simulink model "sensor_model"  (R2018a)
settings: Solver=ode15s  StartTime=0.0  StopTime=200  RelTol=1e-3
libraries: simulink x3
settings Model: Creator=cory0  LastModifiedBy=sanjana

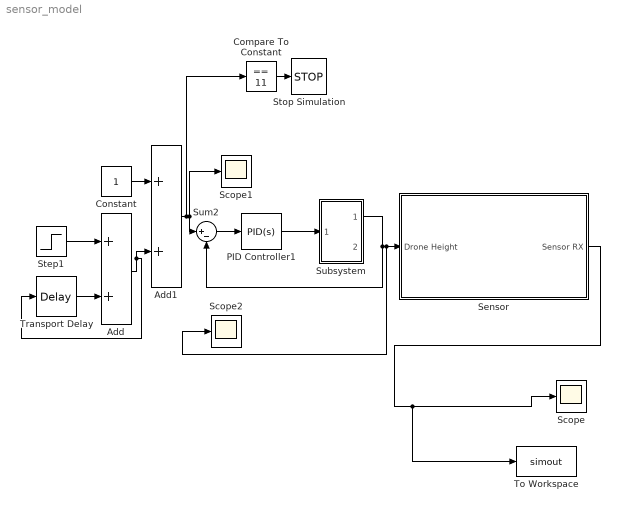
== system sensor_model ==
  Add : Sum
  Add1 : Sum
  Compare To Constant : simulink/Logic and Bit Operations/Compare To Constant  relop===  const=11  OutDataTypeStr=boolean
  Constant : Constant
  PID Controller1 : simulink/Continuous/PID Controller  Controller=PID  TimeDomain=Continuous-time  SampleTime=-1  IntegratorMethod=Forward Euler  FilterMethod=Forward Euler  Form=Parallel  UseFilter=on  ControllerParametersSource=internal  P=85  I=0  D=85  N=10  InitialConditionSource=internal  InitialConditionForIntegrator=0  InitialConditionForFilter=0  ExternalReset=none  LimitOutput=off  UpperSaturationLimit=inf  LowerSaturationLimit=-inf  LinearizeAsGain=on  AntiWindupMode=none  Kb=1  TrackingMode=off  Kt=1  PParamMin=[]  PParamMax=[]  IParamMin=[]  IParamMax=[]  DParamMin=[]  DParamMax=[]  NParamMin=[]  NParamMax=[]  KbParamMin=[]  KbParamMax=[]  KtParamMin=[]  KtParamMax=[]  POutMin=[]  POutMax=[]  IOutMin=[]  IOutMax=[]  DOutMin=[]  DOutMax=[]  NOutMin=[]  NOutMax=[]  KbOutMin=[]  KbOutMax=[]  KtOutMin=[]  KtOutMax=[]  IntegratorOutMin=[]  IntegratorOutMax=[]  FilterOutMin=[]  FilterOutMax=[]  SumOutMin=[]  SumOutMax=[]  SumI1OutMin=[]  SumI1OutMax=[]  SumI2OutMin=[]  SumI2OutMax=[]  SumI3OutMin=[]  SumI3OutMax=[]  SumDOutMin=[]  SumDOutMax=[]  SaturationOutMin=[]  SaturationOutMax=[]  IntegratorContinuousStateAttributes=''  IntegratorStateMustResolveToSignalObject=off  IntegratorRTWStateStorageClass=Auto  FilterContinuousStateAttributes=''  FilterStateMustResolveToSignalObject=off  FilterRTWStateStorageClass=Auto  DifferentiatorICPrevScaledInput=0  DifferentiatorOutMin=[]  DifferentiatorOutMax=[]  FilterDiffOutCoefMin=[]  FilterDiffOutCoefMax=[]  SumDenOutMin=[]  SumDenOutMax=[]  SumNumOutMin=[]  SumNumOutMax=[]  ReciprocalOutMin=[]  ReciprocalOutMax=[]  DivideOutMin=[]  DivideOutMax=[]  TunerSelectOption=Transfer Function Based (PID Tuner App)
  Scope : Scope
  Scope1 : Scope
  Scope2 : Scope
  Sensor : Subsystem
  Step1 : Step  Time=15  SampleTime=0
  Stop Simulation : Stop
  Subsystem : Subsystem
  Sum2 : Sum  Inputs=|+-
  To Workspace : ToWorkspace  VariableName=simout  SampleTime=0.005
  Transport Delay : TransportDelay  DelayTime=20
  wires:
  Constant/1 -> Add1/1
  Subsystem/1(Out1) -> Scope2/1, Sensor/1(Drone Height), Sum2/2
  PID Controller1/1 -> Subsystem/1(In1)
  Sum2/1 -> PID Controller1/1
  Transport Delay/1 -> Add/2
  Step1/1 -> Add/1
  Add1/1 -> Compare To Constant/1, Scope1/1, Sum2/1
  Add/1 -> Transport Delay/1, Add1/2
  Compare To Constant/1 -> Stop Simulation/1
  Sensor/1(Sensor RX) -> To Workspace/1, Scope/1

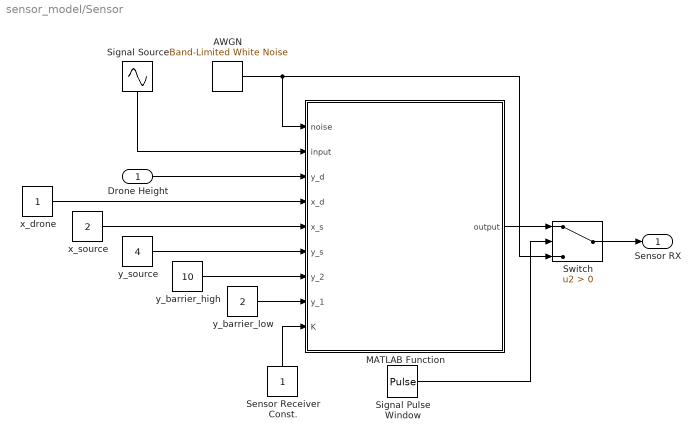
== system sensor_model/Sensor ==
  Drone Height : Inport
  AWGN : simulink/Sources/Band-Limited White Noise  Cov=[0.00001]  Ts=0.0005  seed=[23340]
  MATLAB Function : MATLAB Function  TreatAsAtomicUnit=on
  Sensor Receiver Const. : Constant
  Signal Source : Sin  Amplitude=10  Frequency=6.2831853  SampleTime=0
  Signal Pulse Window : DiscretePulseGenerator  PulseType=Time based  Period=20  PulseWidth=75
  Switch : Switch  Criteria=u2 > Threshold
  x_drone : Constant
  x_source : Constant  Value=2
  y_barrier_high : Constant  Value=10
  y_barrier_low : Constant  Value=2
  y_source : Constant  Value=4
  Sensor RX : Outport
  wires:
  Sensor Receiver Const./1 -> MATLAB Function/9(K)
  Signal Source/1 -> MATLAB Function/2(input)
  Signal Pulse Window/1 -> Switch/2
  y_source/1 -> MATLAB Function/6(y_s)
  y_barrier_low/1 -> MATLAB Function/8(y_1)
  x_drone/1 -> MATLAB Function/4(x_d)
  MATLAB Function/1(output) -> Switch/1
  AWGN/1 -> MATLAB Function/1(noise), Switch/3
  y_barrier_high/1 -> MATLAB Function/7(y_2)
  x_source/1 -> MATLAB Function/5(x_s)
  Drone Height/1 -> MATLAB Function/3(y_d)
  Switch/1 -> Sensor RX/1

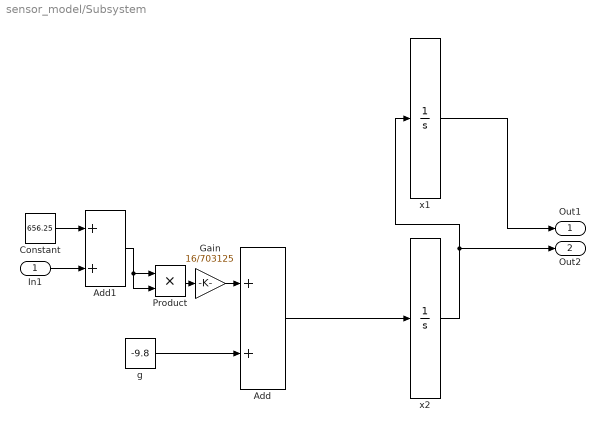
== system sensor_model/Subsystem ==
  In1 : Inport
  Add : Sum
  Add1 : Sum
  Constant : Constant  Value=656.25
  Gain : Gain  Gain=16/703125
  Product : Product
  g : Constant  Value=-9.8
  x1 : Integrator  InitialCondition=0.0000001
  x2 : Integrator
  Out1 : Outport
  Out2 : Outport  Port=2
  wires:
  x2/1 -> Out2/1, x1/1
  x1/1 -> Out1/1
  g/1 -> Add/2
  Add/1 -> x2/1
  Product/1 -> Gain/1
  Gain/1 -> Add/1
  Add1/1 -> Product/2, Product/1
  Constant/1 -> Add1/1
  In1/1 -> Add1/2

== matlab function sensor_model/Sensor/MATLAB Function ==
  data: noise input; input input; y_d input; x_d input; output output; x_s input; y_s input; y_2 input; y_1 input; K input
function output = sensor_filter(noise,input,y_d,x_d,x_s,y_s,y_2,y_1,K)
    
    % Line of Sight Aperture
    c = y_d + (y_s-y_d)*x_d/(x_s+x_d);
    
    % Drone-Sensor Distance
    d = sqrt((x_d+x_s)^2 + (y_d-y_s)^2);
    
    % Sensor Reading
    if (c >= y_1) && (c <= y_2)
        output = sqrt(K)*input/d + noise;
    else
        output = noise;
    end

end
